simulink model "Multi_ToneAMsignal"  (R2019b)
settings: Solver=VariableStepAuto  StartTime=0.0  StopTime=10.0  RelTol=1e-3
libraries: commchan3 x1, commanapbnd3 x1
settings Model: Creator=Kai  LastModifiedBy=Kai

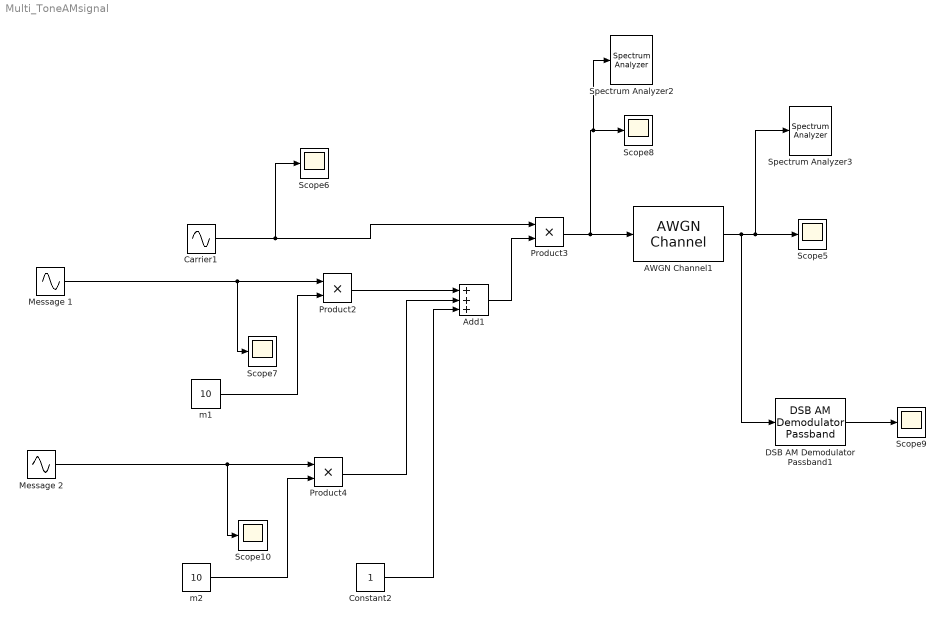
== system Multi_ToneAMsignal ==
  AWGN Channel1 : commchan3/AWGN Channel  InputProcessing=Columns as channels (frame based)  seed=67  noiseMode="Signal to noise ratio  (SNR)"  EbNodB=10  EsNodB=10  SNRdB=3  bitsPerSym=1  Ps=1  Tsym=1  variance=1
      settings: SourceProductName=Communications Toolbox
  Add1 : Sum  Inputs=+++
  Carrier1 : Sin  Frequency=2*pi*25  SampleTime=1/50000
  Constant2 : Constant
  DSB AM Demodulator Passband1 : commanapbnd3/DSB AM Demodulator Passband  Fc=300  Ph=0  method=Butterworth  n=4  cf=300  Rp=0.1  Rs=50  Offset=1
      settings: SourceProductName=Communications Toolbox  SourceProductBaseCode=CM
  Message 1 : Sin  Frequency=2*pi  SampleTime=1/50000
  Message 2 : Sin  Frequency=2*pi  SampleTime=1/50000
  Product2 : Product
  Product3 : Product
  Product4 : Product
  Scope{5..10} (6 alike) : Scope
  Spectrum Analyzer2 : SpectrumAnalyzer
  Spectrum Analyzer3 : SpectrumAnalyzer
  m1 : Constant  Value=10
  m2 : Constant  Value=10
  wires:
  Constant2/1 -> Add1/3
  Message 2/1 -> Scope10/1, Product4/1
  m2/1 -> Product4/2
  DSB AM Demodulator Passband1/1 -> Scope9/1
  Carrier1/1 -> Scope6/1, Product3/1
  AWGN Channel1/1 -> DSB AM Demodulator Passband1/1, Spectrum Analyzer3/1, Scope5/1
  m1/1 -> Product2/2
  Add1/1 -> Product3/2
  Message 1/1 -> Scope7/1, Product2/1
  Product2/1 -> Add1/1
  Product3/1 -> Spectrum Analyzer2/1, Scope8/1, AWGN Channel1/1
  Product4/1 -> Add1/2
